simulink model "AlgoritmiSLX"  (R2023a)
settings: Solver=ode23tb  StartTime=0.0  StopTime=0.1  MaxStep=0.0000001  RelTol=1e-4  AbsTol=1e-4
libraries: simulink x2
settings Model: Creator=gabrielcrisan  LastModifiedBy=gabrielcrisan

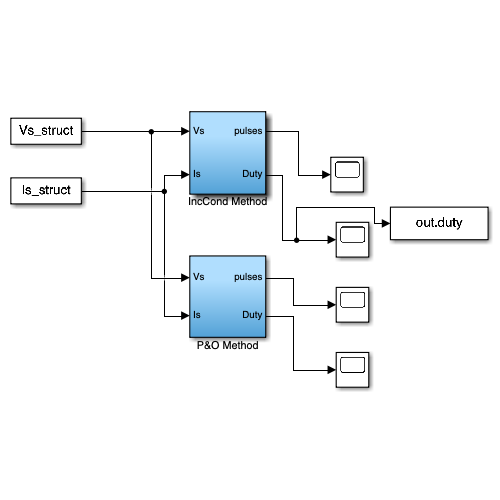
[thumbnail: Simulink's stored preview of the top-level diagram]
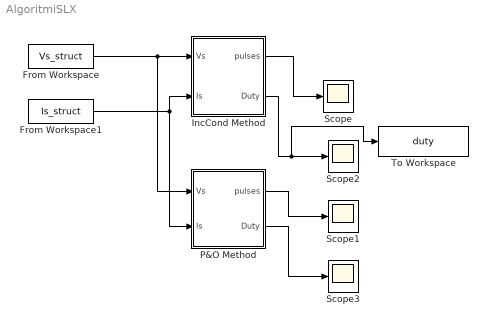
== system AlgoritmiSLX ==
  From Workspace : FromWorkspace  VariableName=Vs_struct
  From Workspace1 : FromWorkspace  VariableName=Is_struct
  IncCond Method : Subsystem  VariantControl=MPPT_IncCond
  P&O Method : Subsystem  VariantControl=MPPT_PandO
  Scope{,1..3} (4 alike) : Scope
  To Workspace : ToWorkspace  VariableName=duty  SaveFormat=Timeseries  SampleTime=-1
  wires:
  From Workspace1/1 -> IncCond Method/2(Is), P&O Method/2(Is)
  From Workspace/1 -> P&O Method/1(Vs), IncCond Method/1(Vs)
  IncCond Method/1(pulses) -> Scope/1
  P&O Method/1(pulses) -> Scope1/1
  IncCond Method/2(Duty) -> To Workspace/1, Scope2/1
  P&O Method/2(Duty) -> Scope3/1

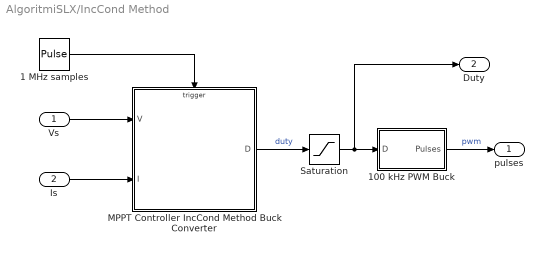
== system AlgoritmiSLX/IncCond Method ==
  Vs : Inport
  Is : Inport  Port=2
  1 MHz samples : DiscretePulseGenerator  PulseType=Time based  Period=0.000001  PulseWidth=5
  100 kHz PWM Buck : Subsystem  mask{Freq=100000}
      mask prompts: Freq "Frequency (Hz)"
  MPPT Controller IncCond Method Buck Converter : Stateflow chart  TreatAsAtomicUnit=on
  Saturation : Saturate  UpperLimit=1  LowerLimit=0  OutMin=[0]  OutMax=[1]
  pulses : Outport
  Duty : Outport  Port=2
  wires:
  Vs/1 -> MPPT Controller IncCond Method Buck Converter/1(V)
  MPPT Controller IncCond Method Buck Converter/1(D) -> Saturation/1  "duty"
  100 kHz PWM Buck/1(Pulses) -> pulses/1  "pwm"
  1 MHz samples/1 -> MPPT Controller IncCond Method Buck Converter/Trigger
  Saturation/1 -> Duty/1, 100 kHz PWM Buck/1(D)
  Is/1 -> MPPT Controller IncCond Method Buck Converter/2(I)

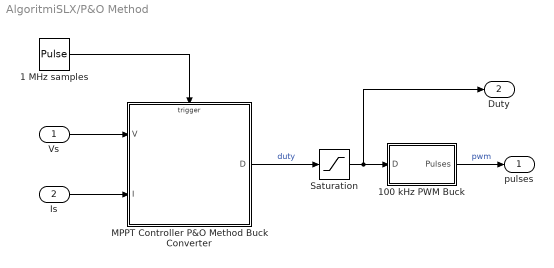
== system AlgoritmiSLX/P&O Method ==
  Vs : Inport
  Is : Inport  Port=2
  1 MHz samples : DiscretePulseGenerator  PulseType=Time based  Period=0.000001  PulseWidth=5
  100 kHz PWM Buck : Subsystem  mask{Freq=100000}
      mask prompts: Freq "Frequency (Hz)"
  MPPT Controller P&O Method Buck Converter : Stateflow chart  TreatAsAtomicUnit=on
  Saturation : Saturate  UpperLimit=1  LowerLimit=0  OutMin=[0]  OutMax=[1]
  pulses : Outport
  Duty : Outport  Port=2
  wires:
  100 kHz PWM Buck/1(Pulses) -> pulses/1  "pwm"
  Is/1 -> MPPT Controller P&O Method Buck Converter/2(I)
  Vs/1 -> MPPT Controller P&O Method Buck Converter/1(V)
  Saturation/1 -> Duty/1, 100 kHz PWM Buck/1(D)
  1 MHz samples/1 -> MPPT Controller P&O Method Buck Converter/Trigger
  MPPT Controller P&O Method Buck Converter/1(D) -> Saturation/1  "duty"

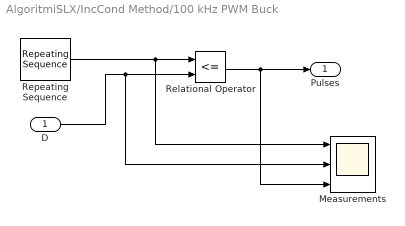
== system AlgoritmiSLX/IncCond Method/100 kHz PWM Buck ==
  D : Inport
  Measurements : Scope  NumInputPorts=3
  Relational Operator : RelationalOperator  Operator=<=  OutDataTypeStr=boolean  ZeroCross=off  InputSameDT=off
  Repeating Sequence : simulink/Sources/Repeating Sequence  rep_seq_t="[0  1/Freq]"  rep_seq_y=[0 1]
  Pulses : Outport
  wires:
  D/1 -> Relational Operator/2, Measurements/2
  Relational Operator/1 -> Pulses/1, Measurements/3
  Repeating Sequence/1 -> Relational Operator/1, Measurements/1

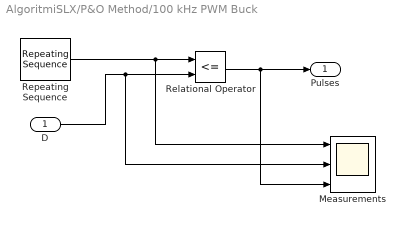
== system AlgoritmiSLX/P&O Method/100 kHz PWM Buck ==
  D : Inport
  Measurements : Scope  NumInputPorts=3
  Relational Operator : RelationalOperator  Operator=<=  OutDataTypeStr=boolean  ZeroCross=off  InputSameDT=off
  Repeating Sequence : simulink/Sources/Repeating Sequence  rep_seq_t="[0  1/Freq]"  rep_seq_y=[0 1]
  Pulses : Outport
  wires:
  Repeating Sequence/1 -> Measurements/1, Relational Operator/1
  Relational Operator/1 -> Measurements/3, Pulses/1
  D/1 -> Measurements/2, Relational Operator/2

== stateflow chart AlgoritmiSLX/IncCond Method/MPPT Controller IncCond Method Buck Converter ==
  state AVERAGE100SAMPLES
    entry:
    Vsum = 0; Isum = 0; k = 0;
    during:
    Vsum = Vsum + V;
    Isum = Isum + I; k++;
    exit:
    Vavg = Vsum/k;
    Iavg = Isum/k;
  state SAMPLEandCALCULATE
    entry:
    deltaV = Vavg - Vprev;
    deltaI = Iavg - Iprev;
    d = D;
  state DECREMENT
    entry:
    d = d - deltad;
  state INCREMENT
    entry:
    d = d + deltad;
  state RETURN
    entry:
    Vprev = Vavg;
    Iprev = Iavg;
    D = d;
  RETURN -> AVERAGE100SAMPLES
  (default) -> AVERAGE100SAMPLES
  AVERAGE100SAMPLES -> SAMPLEandCALCULATE : after(100,clk)
  SAMPLEandCALCULATE -> (junction 16) [order 1] : [deltaV~=0]
  SAMPLEandCALCULATE -> (junction 17) [order 2] : [deltaV==0]
  (junction 17) -> INCREMENT [order 1] : [deltaI < 0]
  (junction 17) -> RETURN [order 3] : [deltaI == 0]
  (junction 16) -> RETURN [order 3] : [deltaI/deltaV == -Iavg/Vavg]
  (junction 16) -> DECREMENT [order 1] : [deltaI/deltaV > -Iavg/Vavg]
  (junction 17) -> DECREMENT [order 2] : [deltaI > 0]
  (junction 16) -> INCREMENT [order 2] : [deltaI/deltaV < -Iavg/Vavg]
  DECREMENT -> RETURN
  INCREMENT -> RETURN
  data: V input; I input; D output double =0.7; k local double; Iavg local double; Iprev local double; Isum local double; Vavg local double; Vprev local double; Vsum local double; d local double; deltaI local double; deltaV local double; deltad local double =8e-3
  events: clk input RISING_EDGE_EVENT

== stateflow chart AlgoritmiSLX/P&O Method/MPPT Controller P&O Method Buck Converter ==
  state AVERAGE100SAMPLES
    entry:
    P = V*I; Psum = 0; Vsum = 0; k = 0;
    during:
    Psum = Psum +P; Vsum = Vsum + V; k++;
    exit:
    Pavg = Psum/k; Vavg = Vsum/k;
  state SAMPLEandCALCULATE
    entry:
    deltaP = Pavg - Pprev;
    deltaV = Vavg - Vprev;
    d = D;
  state DECREMENT
    entry:
    d = d - deltad;
  state INCREMENT
    entry:
    d = d + deltad;
  state RETURN
    entry:
    Pprev = Pavg; Vprev = Vavg; D = d;
  RETURN -> AVERAGE100SAMPLES
  (default) -> AVERAGE100SAMPLES
  AVERAGE100SAMPLES -> SAMPLEandCALCULATE : after(100,clk)
  SAMPLEandCALCULATE -> RETURN [order 1] : [deltaP==0]
  SAMPLEandCALCULATE -> (junction 138) [order 3] : [deltaP < 0]
  SAMPLEandCALCULATE -> (junction 139) [order 2] : [deltaP >0]
  (junction 139) -> INCREMENT [order 1] : [deltaV < 0]
  (junction 138) -> DECREMENT [order 2] : [deltaV < 0]
  (junction 139) -> DECREMENT [order 2] : [deltaV > 0]
  (junction 138) -> INCREMENT [order 1] : [deltaV > 0]
  DECREMENT -> RETURN
  INCREMENT -> RETURN
  data: V input; I input; D output double =0.7; k local double; Vavg local double; Vprev local double; Vsum local double; d local double; deltaV local double; deltad local double =8e-3; P local double; Pavg local double; Pprev local double; Psum local double; deltaP local double
  events: clk input RISING_EDGE_EVENT
